simulink model "sampleModel1402_2_sub"  (R2023a)
settings: Solver=VariableStepAuto  StartTime=0.0  StopTime=10.0  RelTol=1e-3
libraries: hdlsllib x9
settings Model: Creator=user1  LastModifiedBy=user1
settings OptimizationCC: BlockReduction=off  ConditionallyExecuteInputs=off

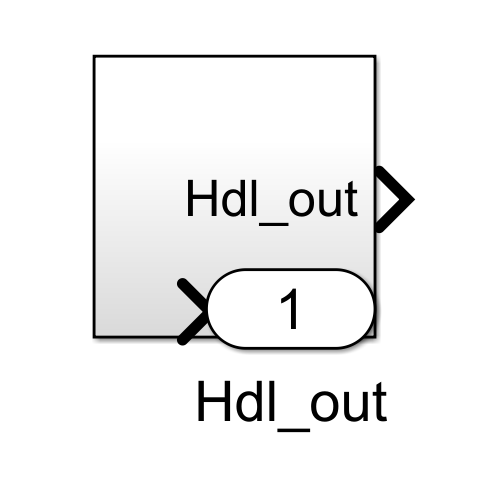
[thumbnail: Simulink's stored preview of the top-level diagram]
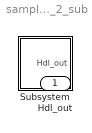
== system sampleModel1402_2_sub ==
  Subsystem : Subsystem
  Hdl_out : Outport  OutDataTypeStr=uint8

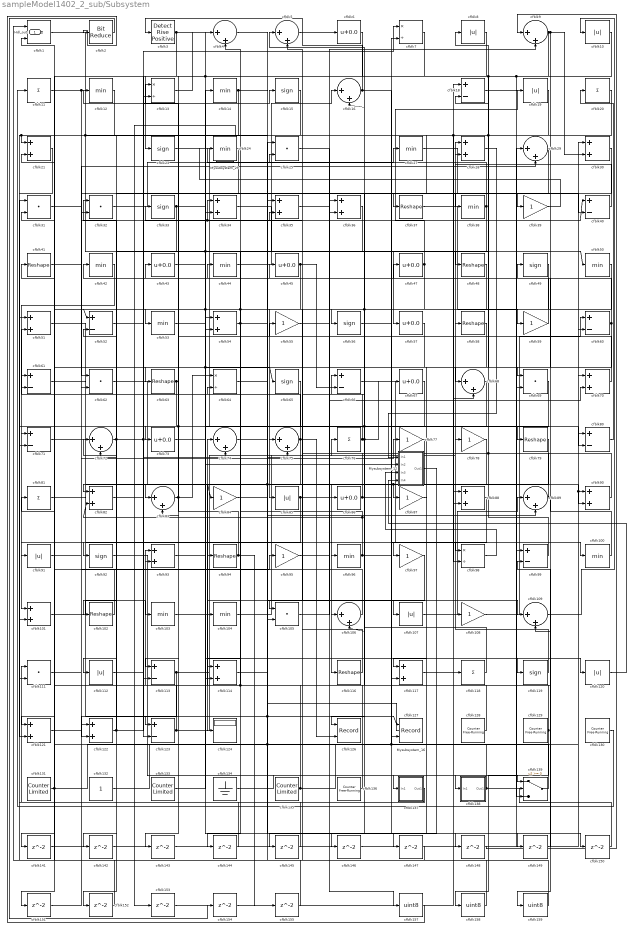
== system sampleModel1402_2_sub/Subsystem ==
  Mysubsystem_12 : Subsystem  TreatAsAtomicUnit=on  RTWFcnName=Mysubsystem_12
      settings: RTWFcnNameOpts=User specified  RTWFileNameOpts=Use function name
  Mysubsystem_16 : Subsystem  TreatAsAtomicUnit=on  RTWFcnName=Mysubsystem_16
      settings: RTWFcnNameOpts=User specified  RTWFileNameOpts=Use function name
  Mysubsystem_29 : Subsystem  TreatAsAtomicUnit=on  RTWFcnName=Mysubsystem_29
      settings: RTWFcnNameOpts=User specified  RTWFileNameOpts=Use function name
  cfblk1 : RelationalOperator  Operator=<=  OutDataTypeStr=boolean  InputSameDT=off
  cfblk{8,10,19,85,91,107,112,120} (8 alike) : Abs  OutDataTypeStr=uint8  SaturateOnIntegerOverflow=off
  cfblk{12,14,24,27,38,42,44,50,53,96,100,103..104} (13 alike) : MinMax  OutDataTypeStr=uint8
  cfblk{21,28,30,34..36,51,54,70,82,88,90,93,101,114,117,121..122} (18 alike) : Sum  OutDataTypeStr=uint8
  cfblk{37,41,48,58,63,79,94,102,116} (9 alike) : Reshape
  cfblk{25,31..32,62,69,105,111} (7 alike) : DotProduct  OutDataTypeStr=uint8
  cfblk{4..5,9,16,29,68,72,74..75,83,89,106,109} (13 alike) : Sum  Inputs=|++  OutDataTypeStr=uint8
  cfblk{39,55,59,77..78,84,87,95,97,108} (10 alike) : Gain  OutDataTypeStr=uint8
  cfblk{11,20,76,81,118} (5 alike) : Sum  Inputs=+  OutDataTypeStr=uint8
  cfblk{18,40,52,60..61,66,71,80,99,113,123} (11 alike) : Sum  Inputs=+-  OutDataTypeStr=uint8
  cfblk{15,23,33,49,56,65,92,119} (8 alike) : Signum
  cfblk124 : Display
  cfblk126 : Record  FileSettingsInternal="{\"entries\":[{\"content\":{\"excelSettings\":{\"content\":{},\"type\":\"Streamout.ExcelSettings\"}},\"type\":\"Streamout.FileSettingStorage\",\"uuid\":\"\"}],\"packageUris\":[\"http:\\/\\/schema.mathworks.com\\/mf0\\/streamout_blocks\\/R2020a\"],\"version\":\"1.0\"}"  Layout=[1 1]  SignalsInternal="{\"entries\":[{\"content\":{\"signals\":[{\"content\":{\"blockPath\":[],\"dimensions\":[1],\"domain\":\"\",\"lineColor\":\"#a2142f\",\"plots\":[1],\"port\":1,\"signalID\":11687,\"signalName\":\"cfblk67\"},\"type\":\"RecordBlkView.Signal\",\"uuid\":\"\"},{\"content\":{\"blockPath\":[],\"dimensions\":[1],\"domain\":\"\",\"lineColor\":\"#139fff\",\"plots\":[1],\"port\":2,\"signalID\":11690,\"signalName\":\"cfblk75\"},\"type\":\"RecordBlkView.Signal\",\"uuid\":\"\"}]},\"type\":\"RecordBlkView.InputSignals\",\"uuid\":\"\"}],\"packageUris\":[\"http:\\/\\/schema.mathworks.com\\/mf0\\/streamout_blocks\\/R2020a\"],\"version\":\"1.0\"}"  VisualizationBindings="{\"xyplotplugin\":{\"info\":[{\"series\":[{\"bindingParametersList\":[{\"parameter\":\"X-Axis\",\"signalID\":11687,\"signalName\":\"cfblk67\"},{\"parameter\":\"Y-Axis\",\"signalID\":11690,\"signalName\":\"cfblk75\"}],\"seriesID\":39533}],\"subplotID\":1}]}}"  CompatibilityTag=XY  st=-1
  cfblk127 : Record  FileSettingsInternal="{\"entries\":[{\"content\":{\"excelSettings\":{\"content\":{},\"type\":\"Streamout.ExcelSettings\"}},\"type\":\"Streamout.FileSettingStorage\",\"uuid\":\"\"}],\"packageUris\":[\"http:\\/\\/schema.mathworks.com\\/mf0\\/streamout_blocks\\/R2020a\"],\"version\":\"1.0\"}"  Layout=[1 1]  SignalsInternal="{\"entries\":[{\"content\":{\"signals\":[{\"content\":{\"blockPath\":[],\"dimensions\":[1],\"domain\":\"\",\"lineColor\":\"#a2142f\",\"plots\":[1],\"port\":1,\"signalID\":11679,\"signalName\":\"cfblk114\"},\"type\":\"RecordBlkView.Signal\",\"uuid\":\"\"},{\"content\":{\"blockPath\":[],\"dimensions\":[1],\"domain\":\"\",\"lineColor\":\"#139fff\",\"plots\":[1],\"port\":2,\"signalID\":11682,\"signalName\":\"cfblk72\"},\"type\":\"RecordBlkView.Signal\",\"uuid\":\"\"}]},\"type\":\"RecordBlkView.InputSignals\",\"uuid\":\"\"}],\"packageUris\":[\"http:\\/\\/schema.mathworks.com\\/mf0\\/streamout_blocks\\/R2020a\"],\"version\":\"1.0\"}"  VisualizationBindings="{\"xyplotplugin\":{\"info\":[{\"series\":[{\"bindingParametersList\":[{\"parameter\":\"X-Axis\",\"signalID\":11679,\"signalName\":\"cfblk114\"},{\"parameter\":\"Y-Axis\",\"signalID\":11682,\"signalName\":\"cfblk72\"}],\"seriesID\":15942}],\"subplotID\":1}]}}"  CompatibilityTag=XY  st=-1
  cfblk{128..130,136} (4 alike) : hdlsllib/Sources/Counter Free-Running  NumBits=16  tsamp=-1
  cfblk{7,13,64,98} (4 alike) : Product  Inputs=*/  OutDataTypeStr=uint8  RndMeth=Zero  SaturateOnIntegerOverflow=on
  cfblk131 : hdlsllib/Sources/Counter Limited  uplimit=7  tsamp=-1
  cfblk132 : Constant  OutDataTypeStr=uint8  SampleTime=-1
  cfblk133 : hdlsllib/Sources/Counter Limited  uplimit=7  tsamp=-1
  cfblk134 : Ground
  cfblk135 : hdlsllib/Sources/Counter Limited  uplimit=7  tsamp=-1
  cfblk137 : Subsystem
      settings: LibrarySourceBlock=|
      | hdlsllib/Ports &
      | Subsystems/Subsystem
  cfblk138 : Subsystem
      settings: LibrarySourceBlock=|
      | hdlsllib/Ports &
      | Subsystems/Subsystem
  cfblk139 : Switch  OutDataTypeStr=uint8  SaturateOnIntegerOverflow=off  InputSameDT=off
  cfblk{141..155} (15 alike) : Delay  SampleTime=1
  cfblk157 : DataTypeConversion  OutDataTypeStr=uint8  SaturateOnIntegerOverflow=off  RndMeth=Floor
  cfblk158 : DataTypeConversion  OutDataTypeStr=uint8  SaturateOnIntegerOverflow=off  RndMeth=Floor
  cfblk159 : DataTypeConversion  OutDataTypeStr=uint8  SaturateOnIntegerOverflow=off  RndMeth=Floor
  cfblk2 : hdlsllib/Logic and Bit Operations/Bit Reduce  mode=AND
  cfblk3 : hdlsllib/Logic and Bit Operations/Detect Rise Positive  vinit=0  OutDataTypeStr=uint8
  cfblk{6,43,45,47,57,67,73,86} (8 alike) : Bias  Bias=0.0  SaturateOnIntegerOverflow=off
  Hdl_out : Outport  OutDataTypeStr=uint8
  wires:
  cfblk51/1 -> cfblk83/1
  cfblk118/1 -> cfblk5/1, cfblk52/1
  cfblk77/1 -> cfblk146/1, cfblk87/1
  cfblk104/1 -> cfblk76/1
  cfblk13/1 -> cfblk4/1
  cfblk44/1 -> cfblk16/1
  cfblk76/1 -> cfblk5/2, cfblk67/1, cfblk16/2
  cfblk37/1 -> cfblk59/1
  cfblk92/1 -> cfblk139/1
  cfblk47/1 -> cfblk106/1, cfblk19/1
  cfblk50/1 -> cfblk53/1
  cfblk138/1(Out1) -> cfblk21/2, cfblk74/1
  cfblk49/1 -> cfblk85/1
  cfblk42/1 -> cfblk101/1
  cfblk3/1 -> cfblk23/1, cfblk50/1, Mysubsystem_12/2(In2)
  cfblk123/1 -> cfblk72/2, cfblk28/1
  cfblk10/1 -> cfblk69/2, cfblk13/2, cfblk68/1
  cfblk23/1 -> cfblk139/2
  cfblk96/1 -> cfblk150/1, cfblk82/2, cfblk44/1
  cfblk116/1 -> cfblk45/1
  cfblk117/1 -> cfblk118/1
  cfblk67/1 -> cfblk126/1
  cfblk31/1 -> cfblk62/1
  cfblk81/1 -> cfblk123/1
  cfblk71/1 -> cfblk97/1
  cfblk103/1 -> cfblk36/1
  cfblk32/1 -> cfblk27/1
  cfblk43/1 -> cfblk120/1, cfblk65/1
  cfblk62/1 -> cfblk116/1
  cfblk108/1 -> cfblk60/1
  cfblk100/1 -> cfblk42/1
  cfblk24/1 -> cfblk123/2
  cfblk15/1 -> cfblk92/1
  cfblk80/1 -> cfblk20/1
  cfblk107/1 -> cfblk89/1
  cfblk1/1 -> cfblk99/1
  cfblk30/1 -> cfblk82/1
  cfblk137/1(Out1) -> cfblk111/1
  cfblk34/1 -> cfblk57/1
  cfblk54/1 -> cfblk107/1, cfblk24/1
  cfblk122/1 -> cfblk52/2, cfblk95/1
  cfblk109/1 -> cfblk10/1
  cfblk11/1 -> cfblk40/2, cfblk75/2, cfblk38/1
  cfblk85/1 -> cfblk98/1, cfblk91/1
  cfblk68/1 -> cfblk106/2, cfblk112/1
  cfblk113/1 -> cfblk122/2, cfblk36/2
  cfblk9/1 -> cfblk141/1, cfblk69/1, cfblk30/2
  cfblk27/1 -> cfblk139/3
  cfblk136/1 -> cfblk93/1
  cfblk130/1 -> cfblk11/1
  cfblk41/1 -> cfblk40/1, cfblk34/1
  cfblk65/1 -> cfblk143/1, cfblk71/2
  cfblk84/1 -> cfblk89/2
  cfblk83/1 -> cfblk64/1, cfblk113/1
  cfblk48/1 -> cfblk105/1
  cfblk90/1 -> cfblk8/1
  cfblk35/1 -> cfblk79/1
  cfblk38/1 -> cfblk114/1, cfblk4/2
  cfblk21/1 -> cfblk101/2
  cfblk16/1 -> cfblk90/2, cfblk3/1
  cfblk20/1 -> cfblk98/2, cfblk37/1
  cfblk139/1 -> cfblk41/1
  cfblk133/1 -> cfblk14/1
  cfblk75/1 -> cfblk104/1, cfblk126/2, cfblk51/2
  cfblk111/1 -> cfblk93/2
  cfblk58/1 -> cfblk117/1
  cfblk12/1 -> cfblk111/2, cfblk21/1
  cfblk73/1 -> cfblk75/1
  cfblk69/1 -> cfblk83/2
  cfblk101/1 -> cfblk103/1
  cfblk78/1 -> cfblk84/1, cfblk105/2
  cfblk40/1 -> cfblk28/2
  cfblk18/1 -> cfblk80/2
  cfblk88/1 -> cfblk117/2
  cfblk61/1 -> cfblk124/1
  cfblk94/1 -> cfblk155/1, cfblk12/1
  cfblk112/1 -> cfblk74/2
  cfblk91/1 -> cfblk29/2
  cfblk131/1 -> cfblk108/1, cfblk61/1
  cfblk86/1 -> cfblk109/1, cfblk55/1
  cfblk102/1 -> cfblk81/1
  cfblk5/1 -> cfblk6/1
  cfblk7/1 -> cfblk73/1
  cfblk128/1 -> cfblk72/1
  cfblk119/1 -> cfblk78/1
  cfblk57/1 -> cfblk121/1
  cfblk74/1 -> cfblk96/1
  cfblk89/1 -> cfblk159/1, cfblk58/1, cfblk33/1
  cfblk66/1 -> cfblk100/1
  cfblk129/1 -> cfblk158/1, cfblk66/1
  cfblk114/1 -> cfblk127/1, cfblk137/1(In1)
  cfblk56/1 -> cfblk119/1
  cfblk45/1 -> cfblk66/2, cfblk94/1, cfblk151/1, cfblk114/2
  cfblk121/1 -> cfblk77/1
  cfblk29/1 -> cfblk56/1
  cfblk72/1 -> cfblk32/1, cfblk127/2, cfblk35/2
  cfblk135/1 -> cfblk88/1, cfblk61/2, cfblk64/2
  cfblk19/1 -> cfblk32/2, cfblk48/1
  cfblk99/1 -> cfblk18/2
  cfblk82/1 -> cfblk7/1
  cfblk52/1 -> cfblk15/1
  cfblk106/1 -> cfblk31/2
  cfblk63/1 -> cfblk13/1, cfblk121/2
  cfblk60/1 -> cfblk63/1, cfblk47/1
  cfblk59/1 -> cfblk49/1
  cfblk14/1 -> cfblk54/2, cfblk88/2
  cfblk55/1 -> cfblk9/2
  cfblk105/1 -> cfblk86/1
  cfblk70/1 -> cfblk43/1
  cfblk8/1 -> cfblk113/2
  cfblk6/1 -> cfblk71/1, cfblk34/2
  cfblk134/1 -> cfblk138/1(In1)
  cfblk95/1 -> cfblk70/2
  cfblk33/1 -> cfblk39/1, cfblk102/1
  cfblk93/1 -> cfblk54/1
  cfblk132/1 -> cfblk35/1, cfblk7/2, cfblk90/1, cfblk60/2
  cfblk141/1 -> cfblk80/1
  cfblk36/1 -> cfblk142/1
  cfblk142/1 -> cfblk29/1
  cfblk143/1 -> cfblk70/1
  cfblk97/1 -> cfblk144/1
  cfblk144/1 -> cfblk51/1
  cfblk145/1 -> cfblk122/1
  cfblk146/1 -> cfblk30/1
  cfblk87/1 -> cfblk147/1
  cfblk147/1 -> cfblk1/1
  cfblk64/1 -> cfblk148/1
  cfblk148/1 -> cfblk9/1
  cfblk53/1 -> cfblk149/1
  cfblk149/1 -> cfblk99/2
  cfblk150/1 -> cfblk109/2
  cfblk151/1 -> cfblk62/2
  cfblk79/1 -> cfblk152/1
  cfblk152/1 -> cfblk31/1
  cfblk153/1 -> cfblk18/1
  cfblk2/1 -> cfblk154/1
  cfblk154/1 -> cfblk68/2
  cfblk155/1 -> cfblk1/2
  cfblk25/1 -> cfblk157/1
  cfblk157/1 -> cfblk2/1
  cfblk158/1 -> cfblk25/1
  cfblk159/1 -> cfblk25/2
  cfblk28/1 -> Mysubsystem_12/1(In1)
  cfblk98/1 -> Mysubsystem_12/3(In3)
  cfblk120/1 -> Mysubsystem_12/4(In4)
  Mysubsystem_12/1(Out1) -> cfblk145/1
  cfblk4/1 -> Mysubsystem_16/1(In1)
  cfblk39/1 -> Mysubsystem_29/1(In1)
  Mysubsystem_29/1(Out1) -> cfblk153/1

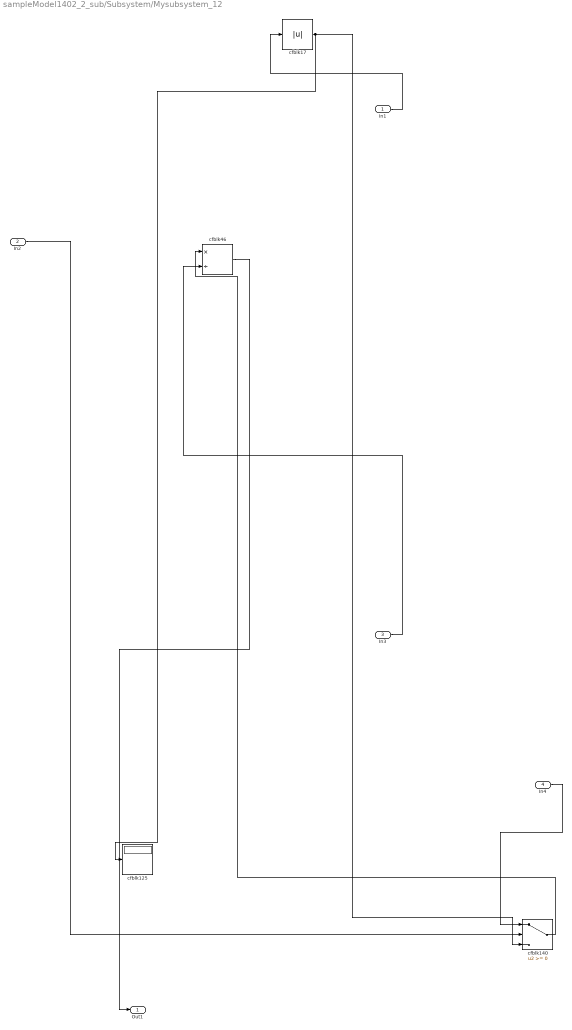
== system sampleModel1402_2_sub/Subsystem/Mysubsystem_12 ==
  In1 : Inport
  In2 : Inport  Port=2
  In3 : Inport  Port=3
  In4 : Inport  Port=4
  cfblk125 : Display
  cfblk140 : Switch  SaturateOnIntegerOverflow=off  InputSameDT=off
  cfblk17 : Abs  SaturateOnIntegerOverflow=off
  cfblk46 : Product  Inputs=*/  RndMeth=Zero  SaturateOnIntegerOverflow=on
  Out1 : Outport
  wires:
  cfblk46/1 -> Out1/1
  In4/1 -> cfblk140/1
  In2/1 -> cfblk140/2
  cfblk17/1 -> cfblk140/3, cfblk125/1
  In1/1 -> cfblk17/1
  In3/1 -> cfblk46/2
  cfblk140/1 -> cfblk46/1

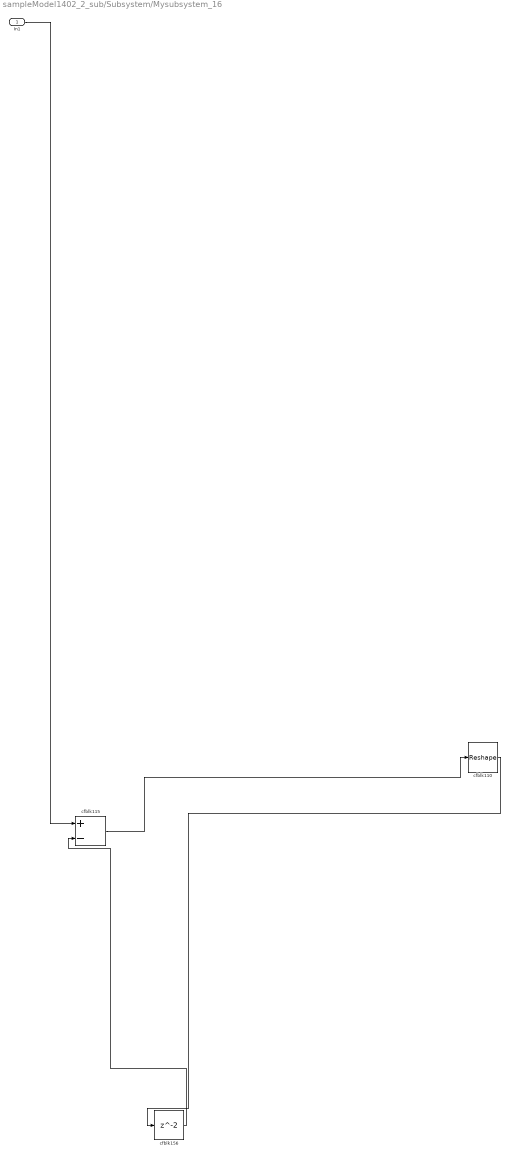
== system sampleModel1402_2_sub/Subsystem/Mysubsystem_16 ==
  In1 : Inport
  cfblk110 : Reshape
  cfblk115 : Sum  Inputs=+-
  cfblk156 : Delay  SampleTime=1
  wires:
  In1/1 -> cfblk115/1
  cfblk115/1 -> cfblk110/1
  cfblk156/1 -> cfblk115/2
  cfblk110/1 -> cfblk156/1

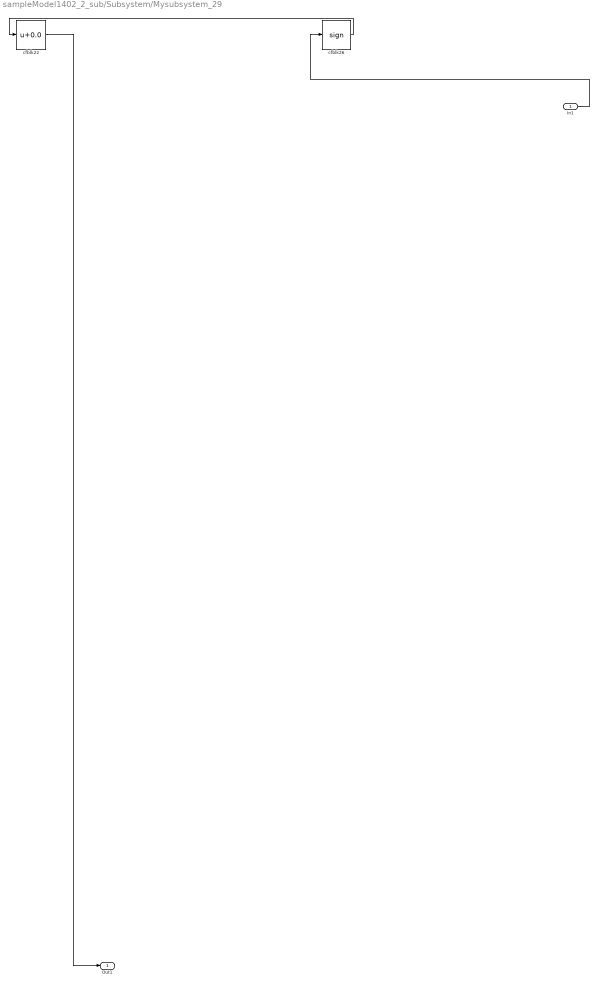
== system sampleModel1402_2_sub/Subsystem/Mysubsystem_29 ==
  In1 : Inport
  cfblk22 : Bias  Bias=0.0  SaturateOnIntegerOverflow=off
  cfblk26 : Signum
  Out1 : Outport
  wires:
  cfblk22/1 -> Out1/1
  In1/1 -> cfblk26/1
  cfblk26/1 -> cfblk22/1

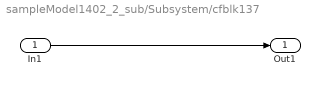
== system sampleModel1402_2_sub/Subsystem/cfblk137 ==
  In1 : Inport
  Out1 : Outport
  wires:
  In1/1 -> Out1/1

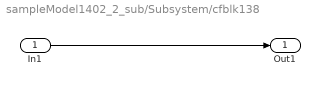
== system sampleModel1402_2_sub/Subsystem/cfblk138 ==
  In1 : Inport
  Out1 : Outport
  wires:
  In1/1 -> Out1/1
